simulink model "p1d1"  (R2023b)
settings: Solver=VariableStepAuto  StartTime=0.0  StopTime=100  RelTol=1e-3
libraries: simulink x1
settings Model: Creator=tanvi  LastModifiedBy=m96sz

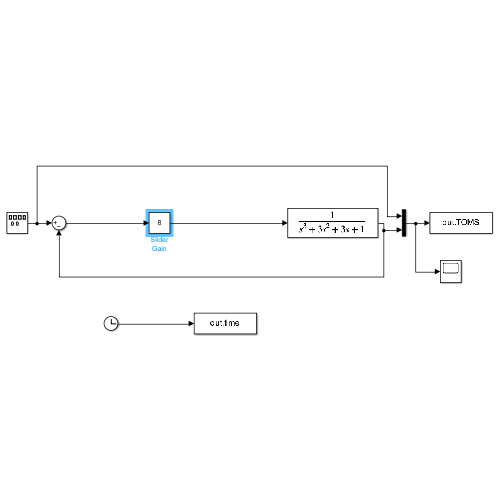
[thumbnail: Simulink's stored preview of the top-level diagram]
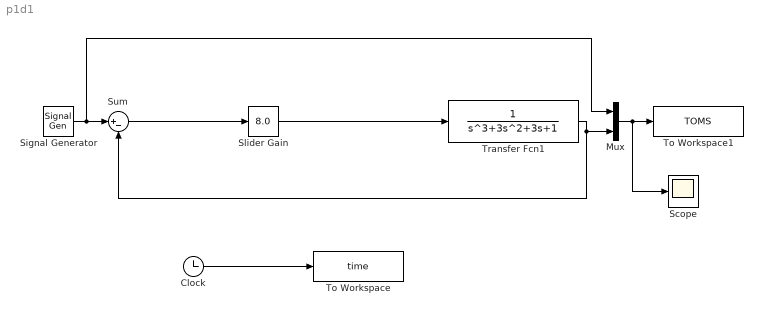
== system p1d1 ==
  Clock : Clock
  Mux : Mux  Inputs=2
  Scope : Scope
  Signal Generator : SignalGenerator  WaveForm=square  Frequency=0.01
  Slider Gain : simulink/Math Operations/Slider Gain  gain=8.0  low=0  high=10
  Sum : Sum  Inputs=|+-
  To Workspace : ToWorkspace  VariableName=time  SampleTime=-1
  To Workspace1 : ToWorkspace  VariableName=TOMS  SampleTime=-1
  Transfer Fcn1 : TransferFcn  Denominator=[1 3 3 1]
  wires:
  Mux/1 -> Scope/1, To Workspace1/1
  Signal Generator/1 -> Mux/1, Sum/1
  Transfer Fcn1/1 -> Sum/2, Mux/2
  Clock/1 -> To Workspace/1
  Sum/1 -> Slider Gain/1
  Slider Gain/1 -> Transfer Fcn1/1
